simulink model "Filter_testaus_uusi"  (R2017b)
settings: Solver=FixedStepDiscrete  StartTime=0.0  StopTime=10  FixedStep=1/44100  RelTol=1e-3
(part 4 of 4)

== system Filter_testaus_uusi/Lowpass/LowpassH/Resonator8 ==
  In1 : Inport
  Constant : Constant  Value=0i
  Delay : Delay  DelayLength=1
  Gain : Gain  Gain=0.97537+0.22058i
  GainH : Gain  Gain=0.6897+0.7241i
  Real-Imag to Complex : RealImagToComplex
  Sum1 : Sum  Inputs=|++
  Out1 : Outport
  wires:
  Constant/1 -> Real-Imag to Complex/2
  In1/1 -> Real-Imag to Complex/1
  Real-Imag to Complex/1 -> Sum1/1
  GainH/1 -> Out1/1
  Gain/1 -> Sum1/2
  Delay/1 -> Gain/1
  Sum1/1 -> Delay/1, GainH/1

== system Filter_testaus_uusi/Lowpass/LowpassH/Resonator9 ==
  In1 : Inport
  Constant : Constant  Value=0i
  Delay : Delay  DelayLength=1
  Gain : Gain  Gain=0.96886+0.24761i
  GainH : Gain  Gain=0.99961+0.027798i
  Real-Imag to Complex : RealImagToComplex
  Sum1 : Sum  Inputs=|++
  Out1 : Outport
  wires:
  Constant/1 -> Real-Imag to Complex/2
  In1/1 -> Real-Imag to Complex/1
  Real-Imag to Complex/1 -> Sum1/1
  GainH/1 -> Out1/1
  Gain/1 -> Sum1/2
  Delay/1 -> Gain/1
  Sum1/1 -> Delay/1, GainH/1

== system Filter_testaus_uusi/Lowpass/LowpassH/ResonatorTemplate ==
  In1 : Inport
  Constant : Constant  Value=0i
  Delay : Delay  DelayLength=1
  Gain : Gain
  GainH : Gain
  Real-Imag to Complex : RealImagToComplex
  Sum1 : Sum  Inputs=|++
  Out1 : Outport
  wires:
  Sum1/1 -> GainH/1, Delay/1
  Delay/1 -> Gain/1
  Gain/1 -> Sum1/2
  GainH/1 -> Out1/1
  Real-Imag to Complex/1 -> Sum1/1
  In1/1 -> Real-Imag to Complex/1
  Constant/1 -> Real-Imag to Complex/2
